simulink model "ComparaMotores"  (R2023b)
settings: Solver=VariableStepAuto  StartTime=0.0  StopTime=10.0  RelTol=1e-3
settings Model: Creator=johan  LastModifiedBy=johan

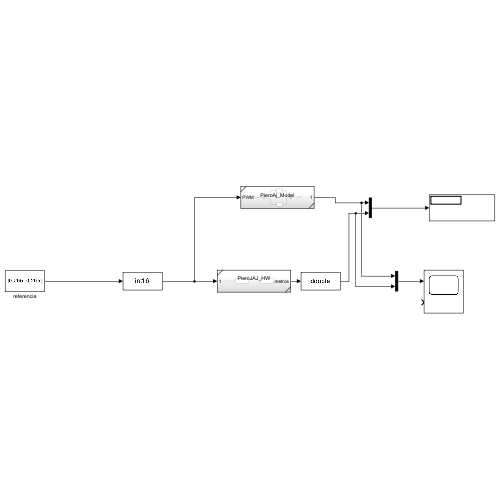
[thumbnail: Simulink's stored preview of the top-level diagram]
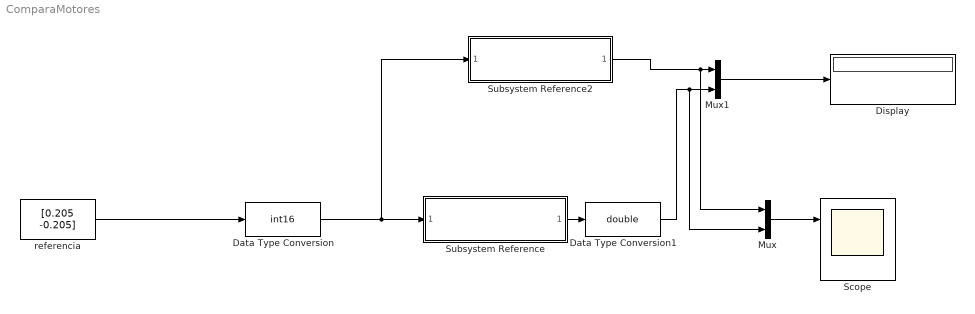
== system ComparaMotores ==
  Data Type Conversion : DataTypeConversion  OutDataTypeStr=int16  SaturateOnIntegerOverflow=off  RndMeth=Floor
  Data Type Conversion1 : DataTypeConversion  OutDataTypeStr=double  SaturateOnIntegerOverflow=off  RndMeth=Floor
  Display : Display
  Mux : Mux  Inputs=2
  Mux1 : Mux  Inputs=2
  Scope : Scope  NumInputPorts=2
  Subsystem Reference : Subsystem  ReferencedSubsystem=PieroJAJ_HW
  Subsystem Reference2 : Subsystem  ReferencedSubsystem=PieroAj_Model
  referencia : Constant  Value=[0.205 -0.205]
  wires:
  Mux1/1 -> Display/1
  Data Type Conversion/1 -> Subsystem Reference/1, Subsystem Reference2/1
  referencia/1 -> Data Type Conversion/1
  Subsystem Reference/1 -> Data Type Conversion1/1
  Subsystem Reference2/1 -> Mux/1, Mux1/1
  Data Type Conversion1/1 -> Mux/2, Mux1/2
  Mux/1 -> Scope/1
